simulink model "Simulation_Block_Diagram_Acceleration"  (R2015b)
settings: Solver=ode45  StartTime=0.0  StopTime=15  FixedStep=1  MaxStep=0.01  MinStep=1e-20  RelTol=1e-4  AbsTol=1e-4
undefined symbols (not defined in the file): A_F, C_0, C_D, F_trac_max, g, G_fd, M_veh, N_r, N_s, P_gen_max, P_mot_max, r_wheel, rho, T_gen_max, T_mot_max, w_eng_max, w_eng_min
libraries: simulink x1
settings Model: Creator=wasynczu  LastModifiedBy=Kane Chew
settings DataIOCC: LimitDataPoints=off  SaveFormat=Array  SignalLoggingSaveFormat=ModelDataLogs
settings OptimizationCC: ExpressionDepthLimit=2147483647
settings DebuggingCC: WriteAfterReadMsg=EnableAllAsError  SolverPrmCheckMsg=warning  FcnCallInpInsideContextMsg=UseLocalSettings  StateNameClashWarn=warning
settings HardwareCC: ProdBitPerPointer=32  ProdLargestAtomicFloat=None  ProdIntDivRoundTo=Undefined  ProdEndianess=Unspecified  ProdWordSize=32  ProdHWDeviceType=32-bit Generic
settings GRTTargetCC: GeneratePreprocessorConditionals=Disable all  CombineOutputUpdateFcns=off  GRTInterface=on
settings ConfigComp: CovModelRefEnable=Off

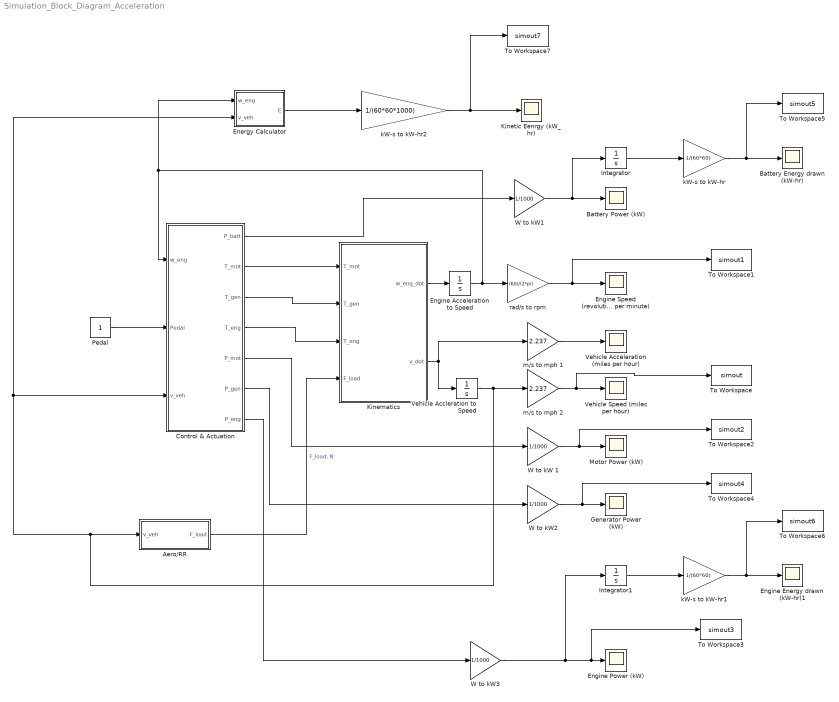
== system Simulation_Block_Diagram_Acceleration ==
  Aero/RR : Subsystem  mask{g=g, M_veh=M_veh, C_drag=C_D, A=A_F, C_rr=C_0, rho=rho}
      mask prompts: g "Earth acceleration, m/s^2"; M_veh "Vehicle mass, kg"; C_drag "Drag coefficient"; A "Frontal area, m^2"; C_rr "Rolling resistance coeeficient"; rho "Air density, kg/m^3"
  Battery Energy drawn (kW-hr) : Scope
  Battery Power (kW) : Scope
  "Control & Actuation " : Subsystem
  Energy Calculator : MATLAB Function  TreatAsAtomicUnit=on
  Engine Acceleration to Speed : Integrator
  Engine Energy drawn (kW-hr)1 : Scope
  Engine Power (kW) : Scope
  Engine Speed (revolutions per minute) : Scope
  Generator Power (kW) : Scope
  Integrator : Integrator
  Integrator1 : Integrator
  Kinematics : MATLAB Function  TreatAsAtomicUnit=on
  Kinetic Eenrgy (kW_hr) : Scope
  Motor Power (kW) : Scope
  Pedal : Constant
  To Workspace : ToWorkspace  VariableName=simout  SaveFormat=Timeseries  SampleTime=-1
  To Workspace1 : ToWorkspace  VariableName=simout1  SaveFormat=Timeseries  SampleTime=-1
  To Workspace2 : ToWorkspace  VariableName=simout2  SaveFormat=Timeseries  SampleTime=-1
  To Workspace3 : ToWorkspace  VariableName=simout3  SaveFormat=Timeseries  SampleTime=-1
  To Workspace4 : ToWorkspace  VariableName=simout4  SaveFormat=Timeseries  SampleTime=-1
  To Workspace5 : ToWorkspace  VariableName=simout5  SaveFormat=Timeseries  SampleTime=-1
  To Workspace6 : ToWorkspace  VariableName=simout6  SaveFormat=Timeseries  SampleTime=-1
  To Workspace7 : ToWorkspace  VariableName=simout7  SaveFormat=Timeseries  SampleTime=-1
  Vehicle Accleration to Speed : Integrator
  Vehicle Acceleration (miles per hour) : Scope
  Vehicle Speed (miles per hour) : Scope
  W to kW 1 : Gain  Gain=1/1000
  W to kW1 : Gain  Gain=1/1000
  W to kW2 : Gain  Gain=1/1000
  W to kW3 : Gain  Gain=1/1000
  kW-s to kW-hr : Gain  Gain=1/(60*60)
  kW-s to kW-hr1 : Gain  Gain=1/(60*60)
  kW-s to kW-hr2 : Gain  Gain=1/(60*60*1000)
  m/s to mph 1 : Gain  Gain=2.237
  m/s to mph 2 : Gain  Gain=2.237
  rad/s to rpm : Gain  Gain=(60)/(2*pi)
  wires:
  Kinematics/2(v_dot) -> m/s to mph 1/1, Vehicle Accleration to Speed/1
  Vehicle Accleration to Speed/1 -> Aero/RR/1(v_veh), Energy Calculator/2(v_veh), "Control & Actuation "/3(v_veh), m/s to mph 2/1
  Aero/RR/1(F_load) -> Kinematics/4(F_load)  "F_load, N"
  Kinematics/1(w_eng_dot) -> Engine Acceleration to Speed/1
  "Control & Actuation "/2(T_mot) -> Kinematics/1(T_mot)
  "Control & Actuation "/3(T_gen) -> Kinematics/2(T_gen)
  "Control & Actuation "/4(T_eng) -> Kinematics/3(T_eng)
  Pedal/1 -> "Control & Actuation "/2(Pedal)
  "Control & Actuation "/1(P_batt) -> W to kW1/1
  m/s to mph 2/1 -> To Workspace/1, Vehicle Speed (miles per hour)/1
  "Control & Actuation "/5("P_mot ") -> W to kW 1/1
  "Control & Actuation "/6(P_gen) -> W to kW2/1
  W to kW 1/1 -> To Workspace2/1, Motor Power (kW)/1
  W to kW2/1 -> To Workspace4/1, Generator Power (kW)/1
  "Control & Actuation "/7(P_eng) -> W to kW3/1
  m/s to mph 1/1 -> Vehicle Acceleration (miles per hour)/1
  Engine Acceleration to Speed/1 -> rad/s to rpm/1, Energy Calculator/1(w_eng), "Control & Actuation "/1("w_eng ")
  rad/s to rpm/1 -> To Workspace1/1, Engine Speed (revolutions per minute)/1
  W to kW1/1 -> Integrator/1, Battery Power (kW)/1
  Integrator/1 -> kW-s to kW-hr/1
  kW-s to kW-hr/1 -> To Workspace5/1, Battery Energy drawn (kW-hr)/1
  W to kW3/1 -> Integrator1/1, To Workspace3/1, Engine Power (kW)/1
  Integrator1/1 -> kW-s to kW-hr1/1
  kW-s to kW-hr1/1 -> To Workspace6/1, Engine Energy drawn (kW-hr)1/1
  Energy Calculator/1(E) -> kW-s to kW-hr2/1
  kW-s to kW-hr2/1 -> To Workspace7/1, Kinetic Eenrgy (kW_hr)/1

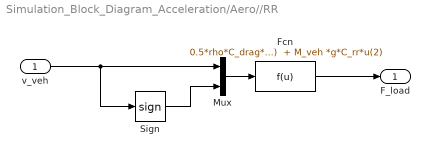
== system Simulation_Block_Diagram_Acceleration/Aero//RR ==
  v_veh : Inport
  Fcn : Fcn  Expr="0.5*rho*C_drag*A*u(1)^2 * u(2)  + M_veh *g*C_rr*u(2)"
  Mux : Mux  Inputs=2
  Sign : Signum  ZeroCross=off
  F_load : Outport
  wires:
  Fcn/1 -> F_load/1
  Mux/1 -> Fcn/1
  v_veh/1 -> Mux/1, Sign/1
  Sign/1 -> Mux/2

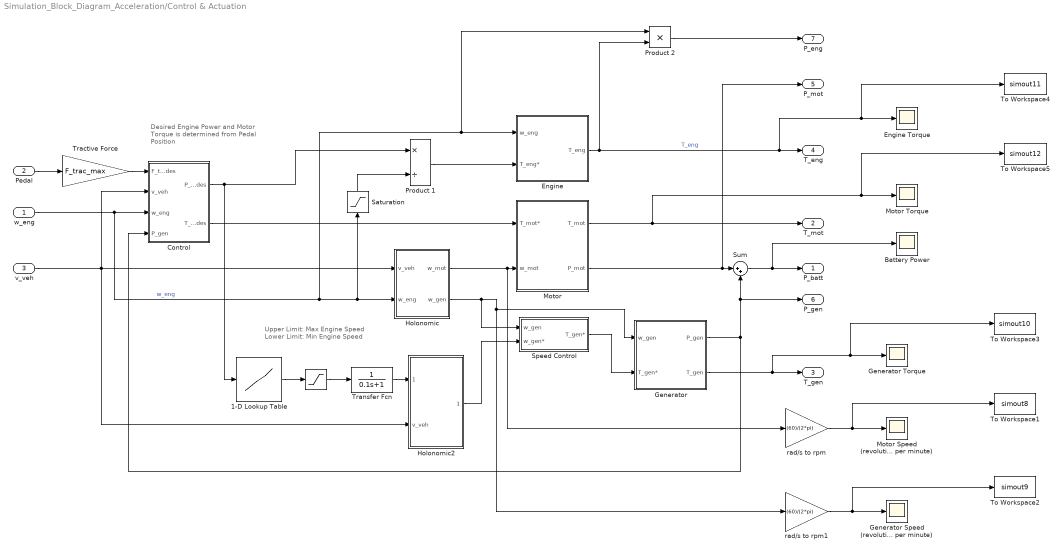
== system Simulation_Block_Diagram_Acceleration/Control & Actuation  ==
  note: Upper Limit: Max Engine Speed
      | Lower Limit: Min Engine Speed
  note: Desired Engine Power and
      | Motor Torque
      | is determined from
      | Pedal Position
  "w_eng " : Inport
  Pedal : Inport  Port=2
  v_veh : Inport  Port=3
  " " : Saturate  UpperLimit=w_eng_max  LowerLimit=w_eng_min
  1-D Lookup Table : Lookup_n-D  NumberOfTableDimensions=1  BreakpointsForDimension1=[1727 2209 2915 4152 5305 5861 6628 7811 8223 9175 10195 14142 19904 26969 35655]  Table=[1178 1172 1160 1166 1178 1166 1172 1184 1172 1184 1281 1688 2210 2830 3510]*(pi/30)  InternalRulePriority=Speed  RndMeth=Simplest  InputSameDT=on
  Battery Power : Scope
  Control : MATLAB Function  TreatAsAtomicUnit=on
  Engine : Subsystem
  Engine Torque : Scope
  Generator : Subsystem
  Generator Speed (revolutions per minute) : Scope
  Generator Torque : Scope
  Holonomic : Subsystem
  Holonomic2 : Subsystem
  Motor : Subsystem
  Motor Speed (revolutions per minute) : Scope
  Motor Torque : Scope
  Product 1 : Product  Inputs=*/
  Product 2 : Product  Inputs=**
  Saturation : Saturate  UpperLimit=inf  LowerLimit=0.01
  Speed Control : Subsystem
  Sum : Sum  Inputs=|++
  To Workspace1 : ToWorkspace  VariableName=simout8  SaveFormat=Timeseries  SampleTime=-1
  To Workspace2 : ToWorkspace  VariableName=simout9  SaveFormat=Timeseries  SampleTime=-1
  To Workspace3 : ToWorkspace  VariableName=simout10  SaveFormat=Timeseries  SampleTime=-1
  To Workspace4 : ToWorkspace  VariableName=simout11  SaveFormat=Timeseries  SampleTime=-1
  To Workspace5 : ToWorkspace  VariableName=simout12  SaveFormat=Timeseries  SampleTime=-1
  Tractive Force : Gain  Gain=F_trac_max
  Transfer Fcn : TransferFcn  Denominator=[0.1 1]
  rad/s to rpm : Gain  Gain=(60)/(2*pi)
  rad/s to rpm1 : Gain  Gain=(60)/(2*pi)
  P_batt : Outport
  T_mot : Outport  Port=2
  T_gen : Outport  Port=3
  T_eng : Outport  Port=4
  "P_mot " : Outport  Port=5
  P_gen : Outport  Port=6
  P_eng : Outport  Port=7
  wires:
  Speed Control/1(T_gen*) -> Generator/2(T_gen*)
  Engine/1(T_eng) -> Product 2/2, To Workspace4/1, Engine Torque/1, T_eng/1  "T_eng"
  Holonomic2/1(w_gen*) -> Speed Control/2(w_gen*)
  Holonomic/1(w_mot) -> rad/s to rpm/1, Motor/2(w_mot)
  Control/2(T_mot_des) -> Motor/1(T_mot*)
  "w_eng "/1 -> Product 2/1, Engine/1(w_eng), Saturation/1, Holonomic/2(w_eng), Control/3(w_eng)  "w_eng"
  Control/1(P_eng_des) -> Product 1/1, 1-D Lookup Table/1
  Saturation/1 -> Product 1/2
  Product 1/1 -> Engine/2(T_eng*)
  Motor/2(P_mot) -> "P_mot "/1, Sum/1
  Generator/1(P_gen) -> P_gen/1, Sum/2, Control/4(P_gen)
  Sum/1 -> Battery Power/1, P_batt/1
  1-D Lookup Table/1 -> " "/1
  Pedal/1 -> Tractive Force/1
  Tractive Force/1 -> Control/1(F_trac_des)
  v_veh/1 -> Holonomic2/2(v_veh), Control/2(v_veh), Holonomic/1(v_veh)
  " "/1 -> Transfer Fcn/1
  Transfer Fcn/1 -> Holonomic2/1(w_eng*)
  Product 2/1 -> P_eng/1
  rad/s to rpm/1 -> To Workspace1/1, Motor Speed (revolutions per minute)/1
  Holonomic/2(w_gen) -> Speed Control/1(w_gen), rad/s to rpm1/1, Generator/1(w_gen)
  rad/s to rpm1/1 -> To Workspace2/1, Generator Speed (revolutions per minute)/1
  Generator/2(T_gen) -> To Workspace3/1, Generator Torque/1, T_gen/1
  Motor/1(T_mot) -> To Workspace5/1, Motor Torque/1, T_mot/1

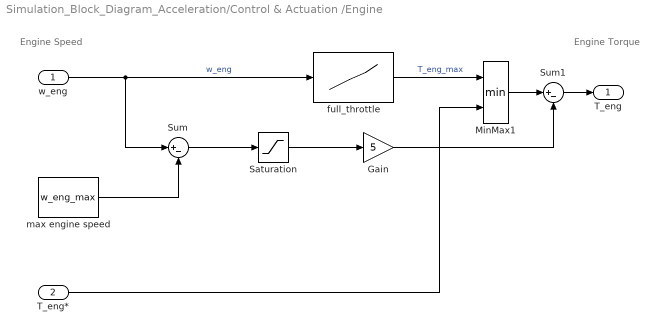
== system Simulation_Block_Diagram_Acceleration/Control & Actuation /Engine ==
  note: Engine Speed
  note: Engine Torque
  w_eng : Inport
  T_eng* : Inport  Port=2
  Gain : Gain  Gain=5
  MinMax1 : MinMax  Inputs=2
  Saturation : Saturate  UpperLimit=inf  LowerLimit=0
  Sum : Sum  Inputs=|+-
  Sum1 : Sum  Inputs=|+-
  full_throttle : Lookup_n-D  NumberOfTableDimensions=1  BreakpointsForDimension1=[1000 1198 1502 1888 2502 3000 3500 4000]*(pi/30)  Table=[76 84 91 97 103 105 107 110]  RndMeth=Simplest  InputSameDT=on
  max engine speed : Constant  Value=w_eng_max
  T_eng : Outport
  wires:
  w_eng/1 -> Sum/1, full_throttle/1  "w_eng"
  T_eng*/1 -> MinMax1/2
  full_throttle/1 -> MinMax1/1  "T_eng_max"
  max engine speed/1 -> Sum/2
  Sum/1 -> Saturation/1
  Sum1/1 -> T_eng/1
  MinMax1/1 -> Sum1/1
  Saturation/1 -> Gain/1
  Gain/1 -> Sum1/2

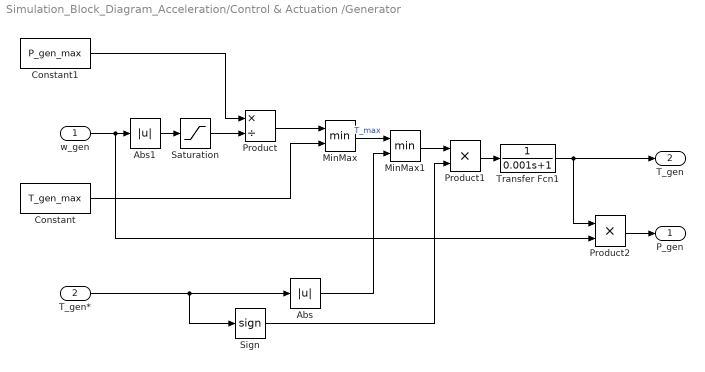
== system Simulation_Block_Diagram_Acceleration/Control & Actuation /Generator ==
  w_gen : Inport
  T_gen* : Inport  Port=2
  Abs : Abs
  Abs1 : Abs
  Constant : Constant  Value=T_gen_max  SampleTime=-1
  Constant1 : Constant  Value=P_gen_max
  MinMax : MinMax  Inputs=2
  MinMax1 : MinMax  Inputs=2
  Product : Product  Inputs=*/
  Product1 : Product
  Product2 : Product
  Saturation : Saturate  UpperLimit=inf  LowerLimit=0.01
  Sign : Signum
  Transfer Fcn1 : TransferFcn  Denominator=[0.001 1]
  P_gen : Outport
  T_gen : Outport  Port=2
  wires:
  w_gen/1 -> Product2/2, Abs1/1
  Saturation/1 -> Product/2
  Product/1 -> MinMax/1
  Constant/1 -> MinMax/2
  Constant1/1 -> Product/1
  MinMax/1 -> MinMax1/1  "T_max"
  T_gen*/1 -> Sign/1, Abs/1
  Abs/1 -> MinMax1/2
  MinMax1/1 -> Product1/1
  Product1/1 -> Transfer Fcn1/1
  Sign/1 -> Product1/2
  Abs1/1 -> Saturation/1
  Transfer Fcn1/1 -> Product2/1, T_gen/1
  Product2/1 -> P_gen/1

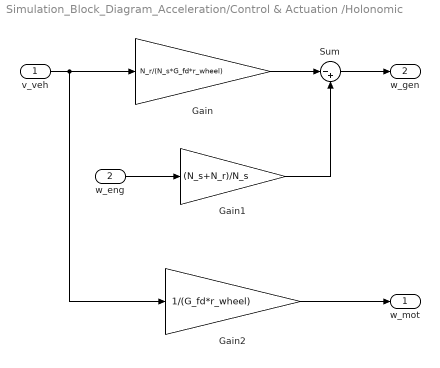
== system Simulation_Block_Diagram_Acceleration/Control & Actuation /Holonomic ==
  v_veh : Inport
  w_eng : Inport  Port=2
  Gain : Gain  Gain=N_r/(N_s*G_fd*r_wheel)
  Gain1 : Gain  Gain=(N_s+N_r)/N_s
  Gain2 : Gain  Gain=1/(G_fd*r_wheel)
  Sum : Sum  Inputs=|-+
  w_mot : Outport
  w_gen : Outport  Port=2
  wires:
  Sum/1 -> w_gen/1
  v_veh/1 -> Gain2/1, Gain/1
  Gain/1 -> Sum/1
  w_eng/1 -> Gain1/1
  Gain1/1 -> Sum/2
  Gain2/1 -> w_mot/1

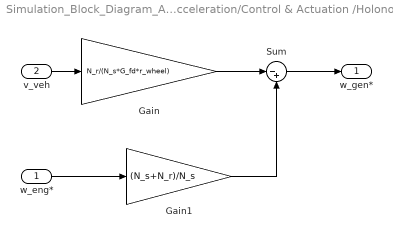
== system Simulation_Block_Diagram_Acceleration/Control & Actuation /Holonomic2 ==
  w_eng* : Inport
  v_veh : Inport  Port=2
  Gain : Gain  Gain=N_r/(N_s*G_fd*r_wheel)
  Gain1 : Gain  Gain=(N_s+N_r)/N_s
  Sum : Sum  Inputs=|-+
  w_gen* : Outport
  wires:
  Sum/1 -> w_gen*/1
  v_veh/1 -> Gain/1
  Gain/1 -> Sum/1
  Gain1/1 -> Sum/2
  w_eng*/1 -> Gain1/1

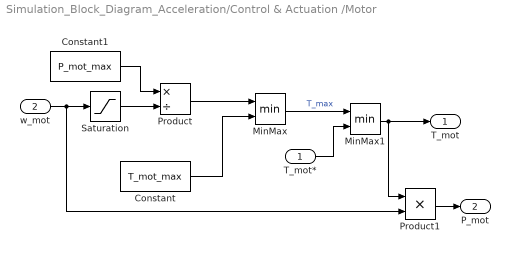
== system Simulation_Block_Diagram_Acceleration/Control & Actuation /Motor ==
  T_mot* : Inport
  w_mot : Inport  Port=2
  Constant : Constant  Value=T_mot_max
  Constant1 : Constant  Value=P_mot_max
  MinMax : MinMax  Inputs=2
  MinMax1 : MinMax  Inputs=2
  Product : Product  Inputs=*/
  Product1 : Product
  Saturation : Saturate  UpperLimit=inf  LowerLimit=0.01
  T_mot : Outport
  P_mot : Outport  Port=2
  wires:
  w_mot/1 -> Product1/2, Saturation/1
  Saturation/1 -> Product/2
  Product/1 -> MinMax/1
  Constant/1 -> MinMax/2
  Constant1/1 -> Product/1
  MinMax/1 -> MinMax1/1  "T_max"
  T_mot*/1 -> MinMax1/2
  MinMax1/1 -> Product1/1, T_mot/1
  Product1/1 -> P_mot/1

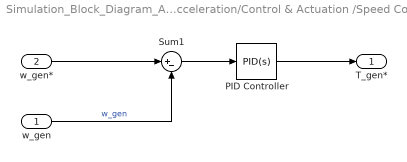
== system Simulation_Block_Diagram_Acceleration/Control & Actuation /Speed Control ==
  w_gen : Inport
  w_gen* : Inport  Port=2
  PID Controller : simulink/Continuous/PID Controller  Controller=PID  TimeDomain=Continuous-time  SampleTime=-1  IntegratorMethod=Forward Euler  FilterMethod=Forward Euler  Form=Parallel  UseFilter=on  ControllerParametersSource=internal  P=100  I=1  D=0  N=100  InitialConditionSource=internal  InitialConditionForIntegrator=0  InitialConditionForFilter=0  ExternalReset=none  LimitOutput=off  UpperSaturationLimit=inf  LowerSaturationLimit=-inf  LinearizeAsGain=on  AntiWindupMode=none  Kb=1  TrackingMode=off  Kt=1  PParamMin=[]  PParamMax=[]  IParamMin=[]  IParamMax=[]  DParamMin=[]  DParamMax=[]  NParamMin=[]  NParamMax=[]  KbParamMin=[]  KbParamMax=[]  KtParamMin=[]  KtParamMax=[]  POutMin=[]  POutMax=[]  IOutMin=[]  IOutMax=[]  DOutMin=[]  DOutMax=[]  NOutMin=[]  NOutMax=[]  KbOutMin=[]  KbOutMax=[]  KtOutMin=[]  KtOutMax=[]  IntegratorOutMin=[]  IntegratorOutMax=[]  FilterOutMin=[]  FilterOutMax=[]  SumOutMin=[]  SumOutMax=[]  SumI1OutMin=[]  SumI1OutMax=[]  SumI2OutMin=[]  SumI2OutMax=[]  SumI3OutMin=[]  SumI3OutMax=[]  SumDOutMin=[]  SumDOutMax=[]  SaturationOutMin=[]  SaturationOutMax=[]  IntegratorContinuousStateAttributes=''  IntegratorStateMustResolveToSignalObject=off  IntegratorRTWStateStorageClass=Auto  FilterContinuousStateAttributes=''  FilterStateMustResolveToSignalObject=off  FilterRTWStateStorageClass=Auto  DifferentiatorICPrevScaledInput=0  DifferentiatorOutMin=[]  DifferentiatorOutMax=[]
  Sum1 : Sum  Inputs=|+-
  T_gen* : Outport
  wires:
  w_gen*/1 -> Sum1/1
  Sum1/1 -> PID Controller/1
  PID Controller/1 -> T_gen*/1
  w_gen/1 -> Sum1/2  "w_gen"

== matlab function Simulation_Block_Diagram_Acceleration/Control & Actuation /Control ==
  data: F_trac_des input; P_eng_des output; v_veh input; T_mot_des output; w_eng input; P_gen input; Param parameter
function [P_eng_des, T_mot_des]  = fcn(F_trac_des, v_veh, w_eng, P_gen, Param)
%#codegen

N_s = Param.N_s;            % number of sun teeth
N_r = Param.N_r;            % number of ring teeth
G_fd = Param.G_fd;
r_wheel = Param.r_wheel;
P_batt_max = Param.P_batt_max; %Assume P_batt = P_batt_max for maximum acceleration
P_eng_max = Param.P_eng_max;

w_gen = w_eng*(N_r+N_s)/N_s - v_veh*N_r/(N_s*G_fd*r_wheel); %Engine Speed
w_mot = v_veh/(G_fd*r_wheel);                               %Motor Speed

%Calculation of Tractive Power
%where F_trac_des = T_mot_max/(G_fd*r_wheel)
P_trac_des = F_trac_des*v_veh;                              

% Condition for Electric Launch
if(P_trac_des < P_batt_max) 
    P_eng_des = 0;                              %Output 1 - Option 1
    T_mot_des = F_trac_des * G_fd * r_wheel;    %Output 2 - Option 2
    return
end

%If P_trac_des > P_batt_max
P_eng_des = P_trac_des - P_batt_max;

%Constraint on Maximum Engine Power
if(P_eng_des > P_eng_max)
    P_eng_des = P_eng_max;                      %Output 1 - Option 2
end

% calculate T_mot_des given P_batt and F_trac

A = [w_gen w_mot; -N_r/(N_s*G_fd*r_wheel) 1/(G_fd*r_wheel)];
b = [P_batt_max; F_trac_des];
x = A\b;
T_mot_des = x(2);                               %Output 2 - Option 2


%Concerning State of Charge
%check to see that P_batt will be less than P_batt_max

P_mot_des = T_mot_des * w_mot;  %Motor Power = Motor Torque * Motor Speed
P_batt_des = P_mot_des + P_gen; %Battery Power = Motor Power + Generator Power

if(P_batt_des > P_batt_max)
   P_mot_des = P_batt_max - P_gen;
   T_mot_des = P_mot_des/w_mot;
end

return

== matlab function Simulation_Block_Diagram_Acceleration/Kinematics ==
  data: T_mot input; T_gen input; T_eng input; Param parameter; w_eng_dot output; F_load input; v_dot output
function [w_eng_dot, v_dot] = fcn(T_mot, T_gen, T_eng, Param,F_load)

N_s = Param.N_s;            %number of sun teeth
N_r = Param.N_r;            %number of ring teeth
G_fd = Param.G_fd;          %differential gear ratio
r_wheel = Param.r_wheel;    %radius of wheel

%Lagrangian Mechanics Equations
%Q_1: Engine
%Q_2: Vehicle
Q_1 = (T_eng + T_gen*(N_s+N_r)/N_s);
Q_2 = (-F_load - T_gen*N_r/N_s/G_fd/r_wheel + T_mot/G_fd/r_wheel);

Q = [Q_1; Q_2]; %Q as a 2 by 1 matrix

%Ay = Q
y = Param.Ainv * Q; 

w_eng_dot = y(1);
v_dot = y(2);

== matlab function Simulation_Block_Diagram_Acceleration/Energy Calculator ==
  data: w_eng input; E output; v_veh input; Param parameter
function E  = fcn(w_eng, v_veh, Param)

J_hat_eng = Param.J_hat_eng;
M_hat_veh = Param.M_hat_veh;
K = Param.K;

%The kinetic energy of the vehicle is calculated as follows
E = (0.5 * J_hat_eng * w_eng * w_eng) + (0.5 * M_hat_veh * v_veh * v_veh) - (K * w_eng * v_veh)

return
